simulink library "sw_lib"  (R2013b)
settings: Solver=ode45  StartTime=0.0  StopTime=10.0  RelTol=1e-3
libraries: simulink x1
settings Model: Creator=raarenst  LastModifiedBy=raarenst

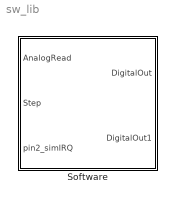
== system sw_lib ==
  Software : Subsystem

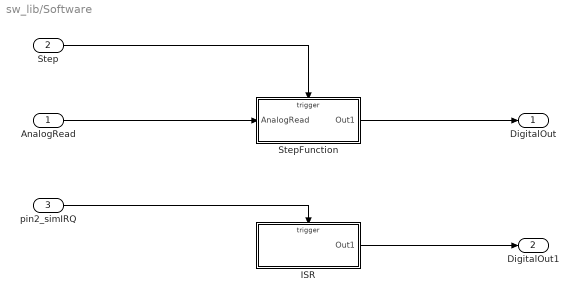
== system sw_lib/Software ==
  AnalogRead : Inport
  Step : Inport  Port=2  OutputFunctionCall=on
  pin2_simIRQ : Inport  Port=3  OutputFunctionCall=on
  ISR : Subsystem  TreatAsAtomicUnit=on
  StepFunction : Subsystem  TreatAsAtomicUnit=on
  DigitalOut : Outport
  DigitalOut1 : Outport  Port=2
  wires:
  Step/1 -> StepFunction/Trigger
  ISR/1(Out1) -> DigitalOut1/1
  pin2_simIRQ/1 -> ISR/Trigger
  StepFunction/1(Out1) -> DigitalOut/1
  AnalogRead/1 -> StepFunction/1(AnalogRead)

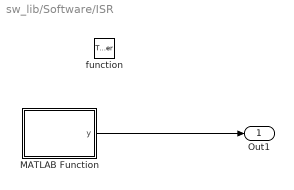
== system sw_lib/Software/ISR ==
  function : TriggerPort  TriggerType=function-call
  MATLAB Function : MATLAB Function  TreatAsAtomicUnit=on
  Out1 : Outport  OutDataTypeStr=boolean  InitialOutput=false
  wires:
  MATLAB Function/1(y) -> Out1/1

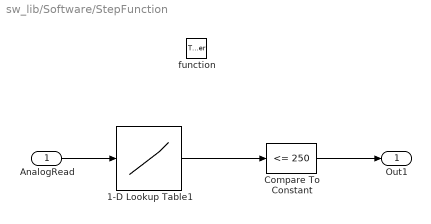
== system sw_lib/Software/StepFunction ==
  AnalogRead : Inport
  function : TriggerPort  TriggerType=function-call
  1-D Lookup Table1 : Lookup_n-D  NumberOfTableDimensions=1  BreakpointsForDimension1=[490 495 500 550 600 650 725 800 900 1050 1250 1550 2000 2550 2750] * 1023/(5*1000)  Table=uint16([150 140 130 120 110 100 90 80 70 60 50 40 30 20 15]*10)  ExtrapMethod=Clip  UseLastTableValue=on  InternalRulePriority=Speed  RndMeth=Simplest  InputSameDT=on
  Compare To Constant : simulink/Logic and Bit Operations/Compare To Constant  relop=<=  const=250  OutDataTypeStr=boolean
  Out1 : Outport  OutDataTypeStr=boolean  InitialOutput=false
  wires:
  Compare To Constant/1 -> Out1/1
  AnalogRead/1 -> 1-D Lookup Table1/1
  1-D Lookup Table1/1 -> Compare To Constant/1

== matlab function sw_lib/Software/ISR/MATLAB Function ==
  data: y output boolean
function y = fcn()
%#codegen

persistent toggle

if isempty(toggle)
    toggle = false;
end

if toggle == false
    toggle = true;
    y = true;
else
   toggle = false;
   y = false;
end
